simulink model "uav_sim_pid"  (R2024a)
settings: Solver=VariableStepAuto  StartTime=0.0  StopTime=60  MaxStep=0.2  RelTol=1e-3
values from neighbouring files (symbols this model uses):
  autopilotParams = block.DialogPrm(1).Data    [autopilot_mpc_sfcn.m]    (also in autopilot_sfcn.m; main_sim_pid.m = NaN(128,1); make_autopilot_parameters_eimpc.m = NaN(128,1))
  gustsNoiseCorrelationTime = 0.5    [make_wind_parameters.m]
  gustsNoisePower = 0.1    [make_wind_parameters.m]
  u_trim = [autopilotParams(28:30); autopilotParams(19)]    [autopilot_sfcn.m]
  uavParams = make_uav_parameters_eimpc()    [main_sim_eimpc.m]    (also in main_sim_pid.m; make_uav_parameters_eimpc.m = NaN(60,1))
  windL = [533 533 533]'    [make_wind_parameters.m]
  windsigma = [3;3;3]    [make_wind_parameters.m]
  windStatic = [-3;2;0]    [make_wind_parameters.m]
undefined symbols (not defined in the file or in its folder): Va0
libraries: simulink x2
settings Model: Creator=piotr  LastModifiedBy=pf
settings RTWCC: GPUComputeCapability=3.5

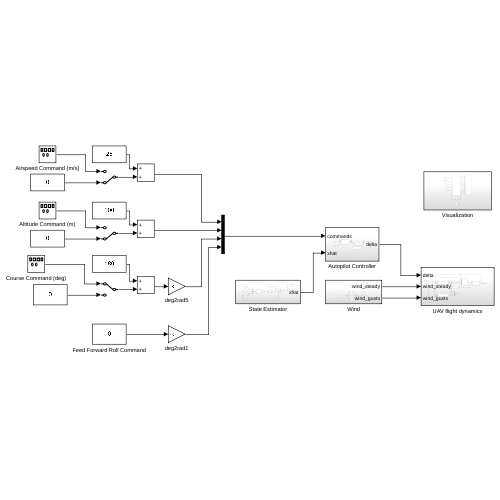
[thumbnail: Simulink's stored preview of the top-level diagram]
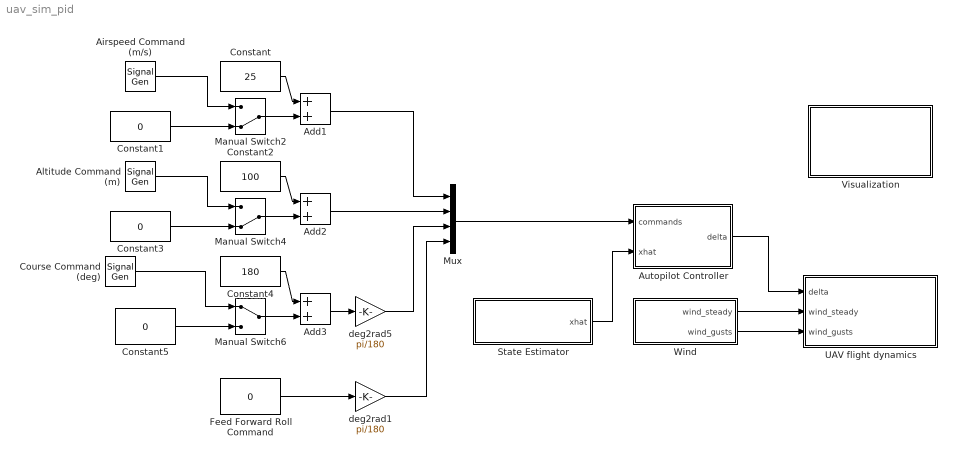
== system uav_sim_pid ==
  Add1 : Sum
  Add2 : Sum
  Add3 : Sum
  Airspeed Command (m/s) : SignalGenerator  WaveForm=square  Amplitude=4  Frequency=0.02
  Altitude Command (m) : SignalGenerator  WaveForm=square  Amplitude=10  Frequency=0.02
  Autopilot Controller : Subsystem
  Constant : Constant  Value=25
  Constant1 : Constant  Value=0
  Constant2 : Constant  Value=100
  Constant3 : Constant  Value=0
  Constant4 : Constant  Value=180
  Constant5 : Constant  Value=0
  Course Command (deg) : SignalGenerator  WaveForm=square  Amplitude=45  Frequency=0.02
  Feed Forward Roll Command : Constant  Value=0
  Manual Switch2 : ManualSwitch  CurrentSetting=0
  Manual Switch4 : ManualSwitch  CurrentSetting=0
  Manual Switch6 : ManualSwitch
  Mux : Mux
  State Estimator : Subsystem
  UAV flight dynamics : Subsystem
  Visualization : Subsystem
  Wind : Subsystem
  deg2rad1 : Gain  Gain=pi/180
  deg2rad5 : Gain  Gain=pi/180
  wires:
  State Estimator/1(xhat) -> Autopilot Controller/2(xhat)
  Wind/2(wind_gusts) -> UAV flight dynamics/3(wind_gusts)
  Wind/1(wind_steady) -> UAV flight dynamics/2(wind_steady)
  Autopilot Controller/1(delta) -> UAV flight dynamics/1(delta)
  deg2rad1/1 -> Mux/4
  Feed Forward Roll Command/1 -> deg2rad1/1
  Altitude Command (m)/1 -> Manual Switch4/1
  Constant2/1 -> Add2/1
  Constant/1 -> Add1/1
  Airspeed Command (m/s)/1 -> Manual Switch2/1
  Add2/1 -> Mux/2
  Manual Switch6/1 -> Add3/2
  Manual Switch2/1 -> Add1/2
  Constant4/1 -> Add3/1
  Manual Switch4/1 -> Add2/2
  Constant5/1 -> Manual Switch6/2
  Add3/1 -> deg2rad5/1
  Mux/1 -> Autopilot Controller/1(commands)
  Course Command (deg)/1 -> Manual Switch6/1
  Constant3/1 -> Manual Switch4/2
  deg2rad5/1 -> Mux/3
  Constant1/1 -> Manual Switch2/2
  Add1/1 -> Mux/1

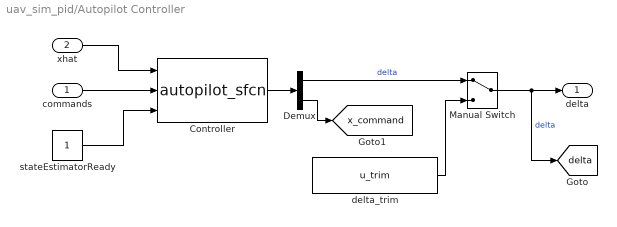
== system uav_sim_pid/Autopilot Controller ==
  commands : Inport
  xhat : Inport  Port=2
  Controller : M-S-Function  FunctionName=autopilot_sfcn  Parameters=autopilotParams
  Demux : Demux  Outputs=[4;12]
  Manual Switch : ManualSwitch
  delta_trim : Constant  Value=u_trim
  stateEstimatorReady : Constant
  delta : Outport
  tag scope: delta=global, x_command=global
  wires:
  Demux/2 -> [x_command]
  Controller/1 -> Demux/1
  xhat/1 -> Controller/1
  stateEstimatorReady/1 -> Controller/3
  commands/1 -> Controller/2
  Manual Switch/1 -> [delta], delta/1  "delta"
  delta_trim/1 -> Manual Switch/2
  Demux/1 -> Manual Switch/1  "delta"

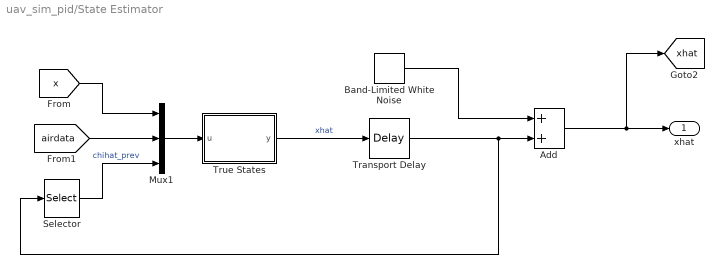
== system uav_sim_pid/State Estimator ==
  Add : Sum
  Band-Limited White Noise : simulink/Sources/Band-Limited White Noise  Cov=autopilotParams(61:79)  Ts=0.1  seed=autopilotParams(81:99)
  Mux1 : Mux  Inputs=[12;6;1]
  Selector : Selector  InputPortWidth=19  IndexOptions=Index vector (dialog)  Indices=[9]  OutputSizes=1
  Transport Delay : TransportDelay  DelayTime=autopilotParams(80)
  True States : MATLAB Function  TreatAsAtomicUnit=on
  xhat : Outport
  tag scope: xhat=global
  wires:
  Band-Limited White Noise/1 -> Add/1
  Add/1 -> [xhat], xhat/1
  True States/1(y) -> Transport Delay/1  "xhat"
  Transport Delay/1 -> Add/2, Selector/1
  [airdata] -> Mux1/2
  Mux1/1 -> True States/1(u)
  [x] -> Mux1/1
  Selector/1 -> Mux1/3  "chihat_prev"

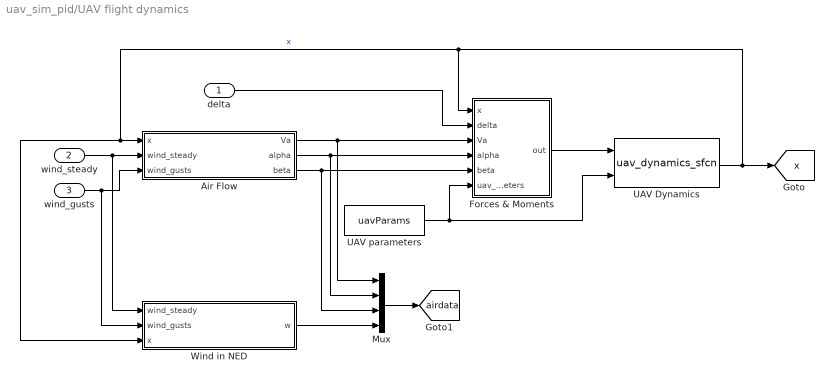
== system uav_sim_pid/UAV flight dynamics ==
  delta : Inport
  wind_steady : Inport  Port=2
  wind_gusts : Inport  Port=3
  Air Flow : MATLAB Function  TreatAsAtomicUnit=on
  Forces & Moments : MATLAB Function  TreatAsAtomicUnit=on
  Mux : Mux
  UAV Dynamics : M-S-Function  FunctionName=uav_dynamics_sfcn  Parameters=x0
  UAV parameters : Constant  Value=uavParams
  Wind in NED : MATLAB Function  TreatAsAtomicUnit=on
  tag scope: airdata=global, x=global
  wires:
  wind_steady/1 -> Wind in NED/1(wind_steady), Air Flow/2(wind_steady)
  wind_gusts/1 -> Wind in NED/2(wind_gusts), Air Flow/3(wind_gusts)
  delta/1 -> Forces & Moments/2(delta)
  Air Flow/1(Va) -> Mux/1, Forces & Moments/3(Va)
  Air Flow/2(alpha) -> Mux/2, Forces & Moments/4(alpha)
  Air Flow/3(beta) -> Mux/3, Forces & Moments/5(beta)
  UAV parameters/1 -> UAV Dynamics/2, Forces & Moments/6(uav_parameters)
  Forces & Moments/1(out) -> UAV Dynamics/1
  UAV Dynamics/1 -> [x], Wind in NED/3(x), Air Flow/1(x), Forces & Moments/1(x)  "x"
  Wind in NED/1(w) -> Mux/4
  Mux/1 -> [airdata]

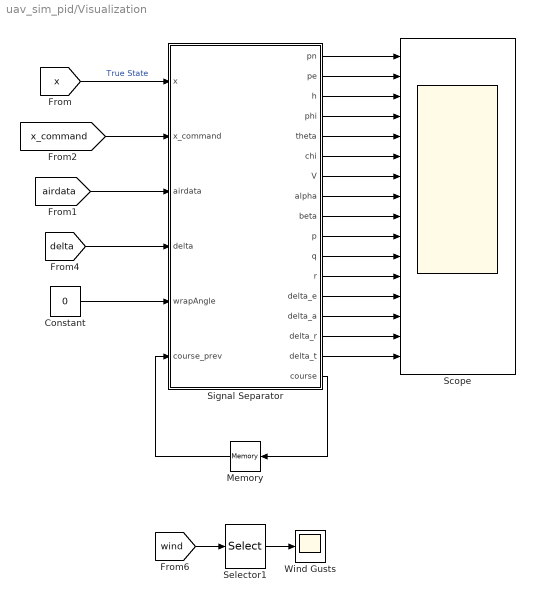
== system uav_sim_pid/Visualization ==
  Constant : Constant  Value=0
  Memory : Memory
  Scope : Scope  NumInputPorts=16
  Selector1 : Selector  InputPortWidth=6  IndexOptions=Index vector (dialog)  Indices=[4 5 6]  OutputSizes=1
  Signal Separator : MATLAB Function  TreatAsAtomicUnit=on
  Wind Gusts : Scope
  wires:
  Signal Separator/16(delta_t) -> Scope/16
  Signal Separator/15(delta_r) -> Scope/15
  Signal Separator/14(delta_a) -> Scope/14
  Signal Separator/13(delta_e) -> Scope/13
  Signal Separator/12(r) -> Scope/12
  Signal Separator/11(q) -> Scope/11
  Signal Separator/10(p) -> Scope/10
  Signal Separator/9(beta) -> Scope/9
  Signal Separator/8(alpha) -> Scope/8
  Signal Separator/7(V) -> Scope/7
  Signal Separator/6(chi) -> Scope/6
  Signal Separator/5(theta) -> Scope/5
  Signal Separator/4(phi) -> Scope/4
  Signal Separator/3(h) -> Scope/3
  Signal Separator/2(pe) -> Scope/2
  Signal Separator/1(pn) -> Scope/1
  [wind] -> Selector1/1
  Selector1/1 -> Wind Gusts/1
  [delta] -> Signal Separator/4(delta)
  [x_command] -> Signal Separator/2(x_command)
  Constant/1 -> Signal Separator/5(wrapAngle)
  Memory/1 -> Signal Separator/6(course_prev)
  Signal Separator/17(course) -> Memory/1
  [airdata] -> Signal Separator/3(airdata)
  [x] -> Signal Separator/1(x)  "True State"

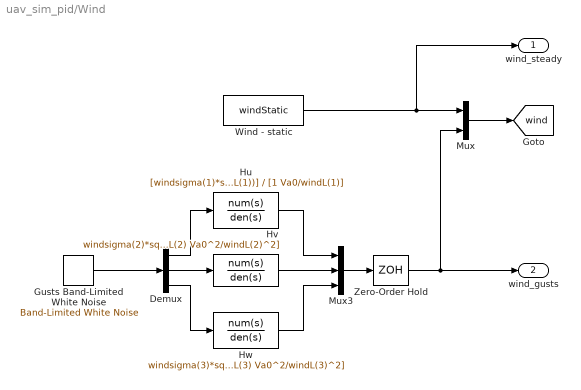
== system uav_sim_pid/Wind ==
  Demux : Demux  Outputs=3
  Gusts Band-Limited White Noise : simulink/Sources/Band-Limited White Noise  Cov=[gustsNoisePower]  Ts=gustsNoiseCorrelationTime  seed=[1 2 3]
  Hu : TransferFcn  Numerator=[windsigma(1)*sqrt(2*Va0/windL(1))]  Denominator=[1 Va0/windL(1)]
  Hv : TransferFcn  Numerator=windsigma(2)*sqrt(3*Va0/windL(2))*[1 Va0/(sqrt(3)*windL(2))]  Denominator=[1 2*Va0/windL(2) Va0^2/windL(2)^2]
  Hw : TransferFcn  Numerator=windsigma(3)*sqrt(3*Va0/windL(3))*[1 Va0/(sqrt(3)*windL(3))]  Denominator=[1 2*Va0/windL(3) Va0^2/windL(3)^2]
  Mux : Mux  Inputs=[3;3]
  Mux3 : Mux  Inputs=3
  Wind - static : Constant  Value=windStatic
  Zero-Order Hold : ZeroOrderHold  SampleTime=-1
  wind_steady : Outport
  wind_gusts : Outport  Port=2
  tag scope: wind=global
  wires:
  Gusts Band-Limited White Noise/1 -> Demux/1
  Demux/3 -> Hw/1
  Demux/1 -> Hu/1
  Demux/2 -> Hv/1
  Zero-Order Hold/1 -> wind_gusts/1, Mux/2
  Mux/1 -> [wind]
  Hu/1 -> Mux3/1
  Mux3/1 -> Zero-Order Hold/1
  Hw/1 -> Mux3/3
  Wind - static/1 -> Mux/1, wind_steady/1
  Hv/1 -> Mux3/2

== matlab function uav_sim_pid/UAV flight dynamics/Air Flow ==
  data: x input; Va output; wind_steady input; wind_gusts input; alpha output; beta output
function [Va, alpha, beta] = fcn(x,wind_steady,wind_gusts)
    [Va, alpha, beta] = airdata(x,wind_steady,wind_gusts);
end

== matlab function uav_sim_pid/State Estimator/True States ==
  data: u input; y output
function y = fcn(u)
    y = true_states(u);
end

== matlab function uav_sim_pid/UAV flight dynamics/Forces & Moments ==
  data: x input; out output; delta input; Va input; alpha input; beta input; uav_parameters input
function out = fcn(x, delta, Va, alpha, beta, uav_parameters)
    out = forces_moments(x, delta, Va, alpha, beta, uav_parameters);
end

== matlab function uav_sim_pid/UAV flight dynamics/Wind in NED ==
  data: wind_steady input; wind_gusts input; x input; w output
function w = fcn(wind_steady,wind_gusts,x)
    w = wind_ned(x,wind_steady,wind_gusts);
end

== matlab function uav_sim_pid/Visualization/Signal Separator ==
  data: x input; pn output; pe output; x_command input; airdata input; h output; phi output; theta output; chi output; V output; alpha output; beta output; p output; q output; r output; delta_e output; delta_a output; delta_r output; delta_t output; delta input; wrapAngle input; course_prev input; course output
function [pn,pe,h,phi,theta,chi,V,alpha,beta,p,q,r,delta_e,delta_a,delta_r,delta_t,course] =...
    fcn(x,x_command,airdata,delta,wrapAngle,course_prev)
    pn = [x(1)];
    pe = [x(2)];
    h = [-x(3); x_command(3)];
    Vg = [norm(x(4:6))];
    phi = [x(7)];
    theta = [x(8)];
    Va_true = airdata(1);
    wn = airdata(4);
    we = airdata(5);
    psi_true = x(9);
    course = atan2(Va_true*sin(psi_true)+we, Va_true*cos(psi_true)+wn);
    course = unwrap_angle(course,course_prev);
    chi = [course; x_command(9); psi_true];
    V = [Va_true; x_command(4); Vg];
    alpha_true = airdata(2);
    beta_true = airdata(3);
    alpha = alpha_true; % TODO [alpha_true; xhat(5)];
    beta = beta_true; % TODO [beta_true; xhat(6)];
    p = [x(10)];
    q = [x(11)];
    r = [x(12)];
    delta(1:3) = rad2deg(delta(1:3));
    delta_e = delta(1);
    delta_a = delta(2);
    delta_r = delta(3);
    delta_t = delta(4);

    phi = rad2deg(phi);
    theta = rad2deg(theta);
    chi = rad2deg(chi);
    alpha = rad2deg(alpha);
    beta = rad2deg(beta);
    p = rad2deg(p);
    q = rad2deg(q);
    r = rad2deg(r);

    if wrapAngle
        phi  = wrapTo180(phi);
        theta = wrapTo180(theta);
        chi = wrapTo180(chi);
        alpha = wrapTo180(alpha);
        beta = wrapTo180(beta);
        delta_e = wrapTo180(delta_e);
        delta_a = wrapTo180(delta_a);
        delta_r = wrapTo180(delta_r);
    end
end
